simulink model "teleop_4ch"  (R2021b)
settings: Solver=VariableStepAuto  StartTime=0.0  StopTime=3  FixedStep=Ts  RelTol=1e-3
undefined symbols (not defined in the file): A, Be, Bh, Bm, Bs, Dh, Dm, Ds, Fc, Flp, Jh, Ke, Km, Ks, Mm, Ms, Ph, xe
settings Model: Creator=fabio  LastModifiedBy=buse

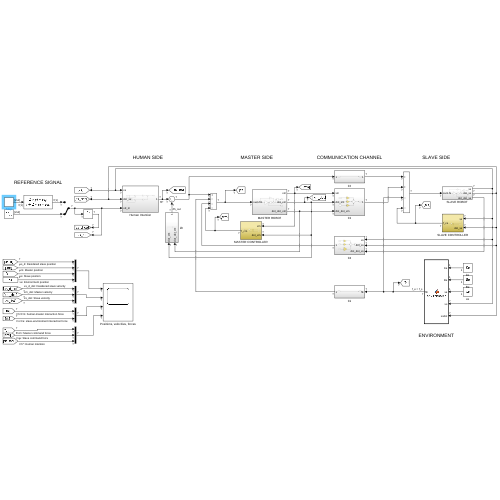
[thumbnail: Simulink's stored preview of the top-level diagram]
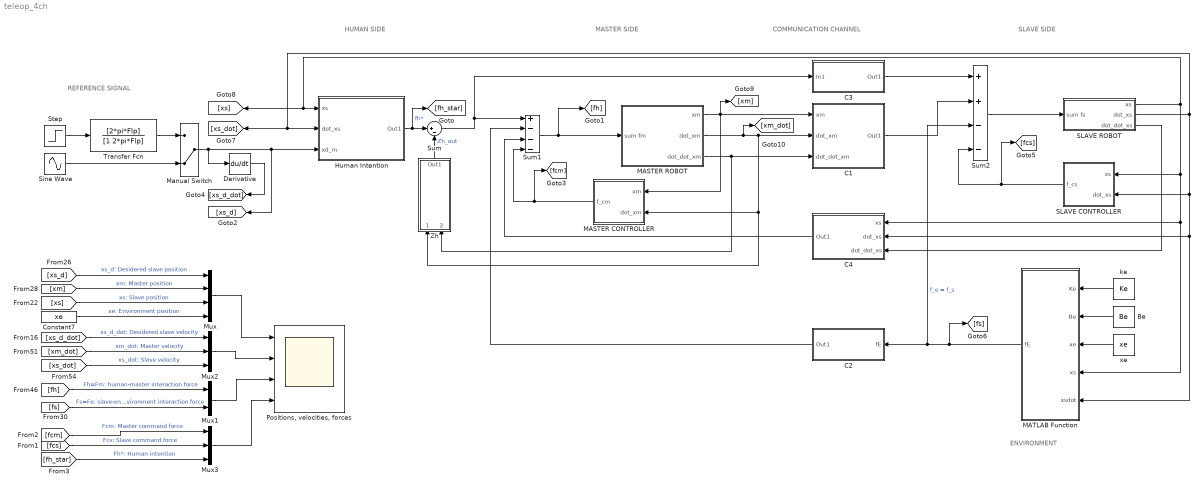
== system teleop_4ch ==
  note: ENVIRONMENT
  note: SLAVE SIDE
  note: COMMUNICATION CHANNEL
  note: MASTER SIDE
  note: HUMAN SIDE
  note: REFERENCE SIGNAL
  Be : Constant  Value=Be
  C1 : Subsystem
  C2 : Subsystem
  C3 : Subsystem
  C4 : Subsystem
  Constant7 : Constant  Value=xe
  Derivative : Derivative
  Human Intention : Subsystem
  MASTER CONTROLLER : Subsystem
  MASTER ROBOT : Subsystem
  MATLAB Function : MATLAB Function  TreatAsAtomicUnit=on
  Manual Switch : ManualSwitch  CurrentSetting=0
  Mux : Mux
  Mux1 : Mux  Inputs=2
  Mux2 : Mux  Inputs=3
  Mux3 : Mux  Inputs=3
  "Positions, velocities, forces" : Scope  NumInputPorts=4
  SLAVE CONTROLLER : Subsystem
  SLAVE ROBOT : Subsystem
  Sine Wave : Sin  Amplitude=A  Frequency=Fc*2*pi  SampleTime=0
  Step : Step  After=A  SampleTime=0
  Sum : Sum  Inputs=|+-
  Sum1 : Sum  Inputs=+---
  Sum2 : Sum  Inputs=++--
  Transfer Fcn : TransferFcn  Numerator=[2*pi*Flp]  Denominator=[1 2*pi*Flp]
  Zh : Subsystem
  ke : Constant  Value=Ke
  xe : Constant  Value=xe
  wires:
  [xs] -> Mux/3  "xs: Slave position"
  Constant7/1 -> Mux/4  "xe: Environment position"
  [xm_dot] -> Mux2/2  "xm_dot: Master velocity"
  Mux2/1 -> "Positions, velocities, forces"/2
  [xs_dot] -> Mux2/3  "xs_dot: Slave velocity"
  [xs_d] -> Mux/1  "xs_d: Desidered slave position"
  [fh] -> Mux1/1  "Fh=Fm: human-master interaction force"
  [xs_d_dot] -> Mux2/1  "xs_d_dot: Desidered slave velocity"
  [xm] -> Mux/2  "xm: Master position"
  [fs] -> Mux1/2  "Fs=Fe: slave-environment interaction force"
  Mux/1 -> "Positions, velocities, forces"/1
  Transfer Fcn/1 -> Manual Switch/1
  Step/1 -> Transfer Fcn/1
  Manual Switch/1 -> Derivative/1, Human Intention/3(xd_m), [xs_d]
  Derivative/1 -> [xs_d_dot]
  Sine Wave/1 -> Manual Switch/2
  [fcm] -> Mux3/1  "Fcm: Master command force"
  [fcs] -> Mux3/2  "Fcs: Slave command force"
  Mux1/1 -> "Positions, velocities, forces"/3
  Mux3/1 -> "Positions, velocities, forces"/4
  [fh_star] -> Mux3/3  "Fh*: Human intention"
  Human Intention/1(Out1) -> [fh_star], Sum/1  "fh*"
  Zh/1(Out1) -> Sum/2  "Zh_out"
  MASTER ROBOT/3(dot_dot_xm) -> C1/3(dot_dot_xm), Zh/2(dot_dot_xm)
  MASTER ROBOT/2(dot_xm) -> Zh/1(dot_xm), MASTER CONTROLLER/2(dot_xm), C1/2(dot_xm), [xm_dot]
  MASTER ROBOT/1(xm) -> [xm], C1/1(xm), MASTER CONTROLLER/1(xm)
  Sum/1 -> C3/1(In1), Sum1/1
  MASTER CONTROLLER/1(f_cm) -> [fcm], Sum1/4
  C2/1(Out1) -> Sum1/2
  C4/1(Out1) -> Sum1/3
  C3/1(Out1) -> Sum2/1
  C1/1(Out1) -> Sum2/2
  xe/1 -> MATLAB Function/3(xe)
  Be/1 -> MATLAB Function/2(Be)
  ke/1 -> MATLAB Function/1(Ke)
  MATLAB Function/1(fE) -> [fs], Sum2/3, C2/1(fE)  "f_e = f_s"
  SLAVE CONTROLLER/1(f_cs) -> Sum2/4, [fcs]
  SLAVE ROBOT/1(xs) -> C4/1(xs), MATLAB Function/4(xs), SLAVE CONTROLLER/1(xs), Human Intention/1(xs), [xs]
  SLAVE ROBOT/2(dot_xs) -> MATLAB Function/5(xsdot), C4/2(dot_xs), SLAVE CONTROLLER/2(dot_xs), Human Intention/2(dot_xs), [xs_dot]
  Sum2/1 -> SLAVE ROBOT/1(sum fs)
  SLAVE ROBOT/3(dot_dot_xs) -> C4/3(dot_dot_xs)
  Sum1/1 -> MASTER ROBOT/1(sum fm), [fh]

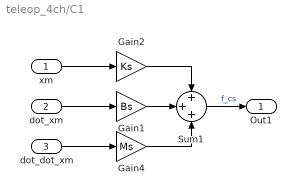
== system teleop_4ch/C1 ==
  xm : Inport
  dot_xm : Inport  Port=2
  dot_dot_xm : Inport  Port=3
  Gain1 : Gain  Gain=Bs
  Gain2 : Gain  Gain=Ks
  Gain4 : Gain  Gain=Ms
  Sum1 : Sum  Inputs=+++
  Out1 : Outport
  wires:
  Gain1/1 -> Sum1/2
  Gain2/1 -> Sum1/1
  xm/1 -> Gain2/1
  dot_xm/1 -> Gain1/1
  Sum1/1 -> Out1/1  "f_cs"
  dot_dot_xm/1 -> Gain4/1
  Gain4/1 -> Sum1/3

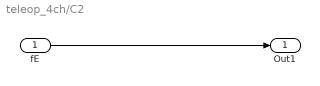
== system teleop_4ch/C2 ==
  fE : Inport
  Out1 : Outport
  wires:
  fE/1 -> Out1/1

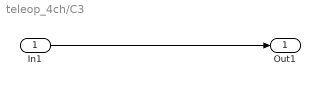
== system teleop_4ch/C3 ==
  In1 : Inport
  Out1 : Outport
  wires:
  In1/1 -> Out1/1

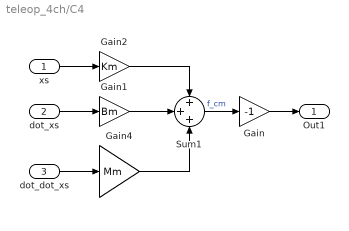
== system teleop_4ch/C4 ==
  xs : Inport
  dot_xs : Inport  Port=2
  dot_dot_xs : Inport  Port=3
  Gain : Gain  Gain=-1
  Gain1 : Gain  Gain=Bm
  Gain2 : Gain  Gain=Km
  Gain4 : Gain  Gain=Mm
  Sum1 : Sum  Inputs=+++
  Out1 : Outport
  wires:
  Gain1/1 -> Sum1/2
  Gain2/1 -> Sum1/1
  xs/1 -> Gain2/1
  dot_xs/1 -> Gain1/1
  Sum1/1 -> Gain/1  "f_cm"
  Gain/1 -> Out1/1
  dot_dot_xs/1 -> Gain4/1
  Gain4/1 -> Sum1/3

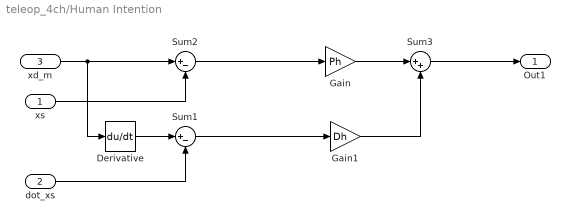
== system teleop_4ch/Human Intention ==
  xs : Inport
  dot_xs : Inport  Port=2
  xd_m : Inport  Port=3
  Derivative : Derivative
  Gain : Gain  Gain=Ph
  Gain1 : Gain  Gain=Dh
  Sum1 : Sum  Inputs=|+-
  Sum2 : Sum  Inputs=|+-
  Sum3 : Sum  Inputs=|++
  Out1 : Outport
  wires:
  xs/1 -> Sum2/2
  dot_xs/1 -> Sum1/2
  Sum2/1 -> Gain/1
  Sum1/1 -> Gain1/1
  Gain1/1 -> Sum3/2
  Gain/1 -> Sum3/1
  Sum3/1 -> Out1/1
  xd_m/1 -> Derivative/1, Sum2/1
  Derivative/1 -> Sum1/1

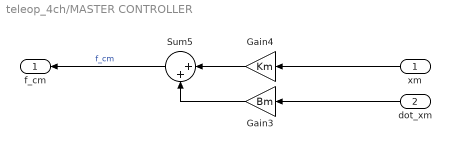
== system teleop_4ch/MASTER CONTROLLER ==
  xm : Inport
  dot_xm : Inport  Port=2
  Gain3 : Gain  Gain=Bm
  Gain4 : Gain  Gain=Km
  Sum5 : Sum  Inputs=|++
  f_cm : Outport
  wires:
  Gain4/1 -> Sum5/1
  Gain3/1 -> Sum5/2
  dot_xm/1 -> Gain3/1
  Sum5/1 -> f_cm/1  "f_cm"
  xm/1 -> Gain4/1

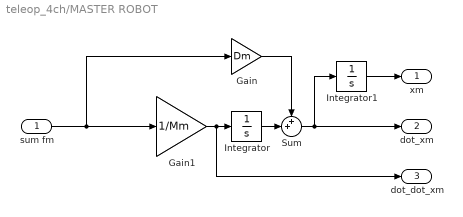
== system teleop_4ch/MASTER ROBOT ==
  sum fm : Inport
  Gain : Gain  Gain=Dm
  Gain1 : Gain  Gain=1/Mm
  Integrator : Integrator
  Integrator1 : Integrator
  Sum : Sum  Inputs=++|
  xm : Outport
  dot_xm : Outport  Port=2
  dot_dot_xm : Outport  Port=3
  wires:
  sum fm/1 -> Gain/1, Gain1/1
  Gain1/1 -> dot_dot_xm/1, Integrator/1
  Sum/1 -> Integrator1/1, dot_xm/1
  Integrator1/1 -> xm/1
  Gain/1 -> Sum/1
  Integrator/1 -> Sum/2

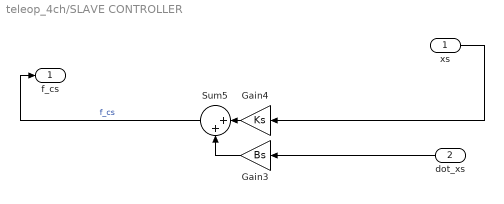
== system teleop_4ch/SLAVE CONTROLLER ==
  xs : Inport
  dot_xs : Inport  Port=2
  Gain3 : Gain  Gain=Bs
  Gain4 : Gain  Gain=Ks
  Sum5 : Sum  Inputs=|++
  f_cs : Outport
  wires:
  Gain4/1 -> Sum5/1
  Gain3/1 -> Sum5/2
  dot_xs/1 -> Gain3/1
  Sum5/1 -> f_cs/1  "f_cs"
  xs/1 -> Gain4/1

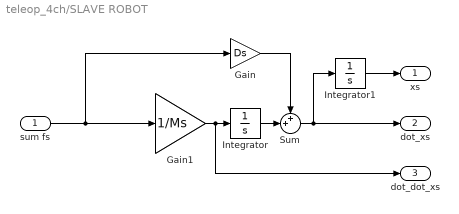
== system teleop_4ch/SLAVE ROBOT ==
  sum fs : Inport
  Gain : Gain  Gain=Ds
  Gain1 : Gain  Gain=1/Ms
  Integrator : Integrator
  Integrator1 : Integrator
  Sum : Sum  Inputs=++|
  xs : Outport
  dot_xs : Outport  Port=2
  dot_dot_xs : Outport  Port=3
  wires:
  sum fs/1 -> Gain/1, Gain1/1
  Gain/1 -> Sum/1
  Sum/1 -> Integrator1/1, dot_xs/1
  Integrator/1 -> Sum/2
  Gain1/1 -> dot_dot_xs/1, Integrator/1
  Integrator1/1 -> xs/1

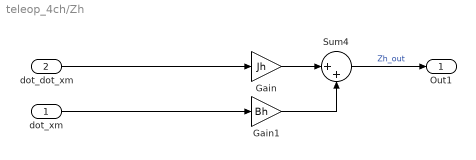
== system teleop_4ch/Zh ==
  dot_xm : Inport
  dot_dot_xm : Inport  Port=2
  Gain : Gain  Gain=Jh
  Gain1 : Gain  Gain=Bh
  Sum4 : Sum  Inputs=|++
  Out1 : Outport
  wires:
  dot_dot_xm/1 -> Gain/1
  Gain1/1 -> Sum4/2
  Gain/1 -> Sum4/1
  Sum4/1 -> Out1/1  "Zh_out"
  dot_xm/1 -> Gain1/1

== matlab function teleop_4ch/MATLAB Function ==
  data: Ke input; fE output; Be input; xe input; xs input; xsdot input
function fE = environment(Ke, Be, xe, xs, xsdot)
    if xs > xe
        fE = Ke * (xs - xe) + Be * xsdot; % Plot both contributions Ke and Be
    else
        fE = 0;
    end
end
